simulink model "Sim_HOSMD"  (R2021a)
settings: Solver=VariableStepAuto  StartTime=ti  StopTime=tf  RelTol=1e-3
values from neighbouring files (symbols this model uses):
  a = 2    [InitParams.m]
  k = 1    [InitParams.m]
  omega = 2    [InitParams.m]
undefined symbols (not defined in the file or in its folder): Noise
libraries: simulink x1
settings Model: Creator=perruquetti  LastModifiedBy=perruquetti
settings SolverCC: AlgebraicLoopSolver=TrustRegion
settings DataIOCC: ReturnWorkspaceOutputs=off
settings DebuggingCC: SFMachineParentedDataDiag=warning  ArithmeticOperatorsInVariantConditions=warning
settings SFSimCC: SimUseLocalCustomCode=off  CustomCodeUndefinedFunction=UseInterfaceOnly
settings RTWCC: RTWUseLocalCustomCode=off

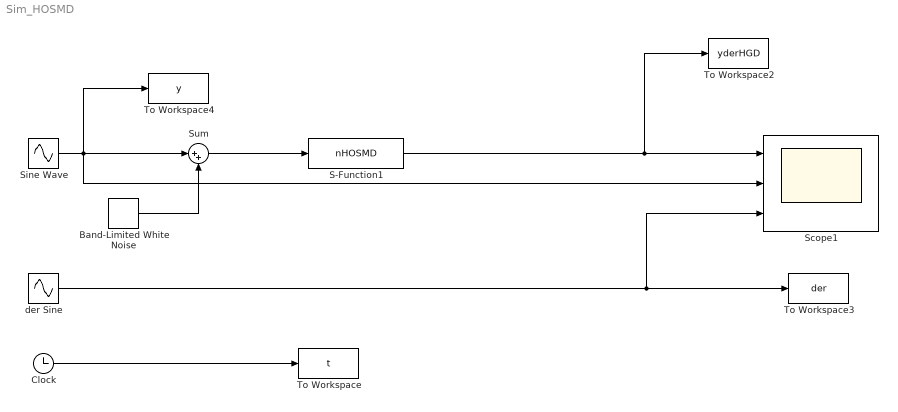
== system Sim_HOSMD ==
  Band-Limited White Noise : simulink/Sources/Band-Limited White Noise  Cov=Noise.power  Ts=Noise.sampling  seed=Noise.seed
  Clock : Clock
  S-Function1 : S-Function  FunctionName=nHOSMD  Parameters=paramsnHOSMD  SFunctionDeploymentMode=off  EnableBusSupport=off
  Scope1 : Scope  NumInputPorts=3
  Sine Wave : Sin  Amplitude=a  Frequency=omega  SampleTime=0
  Sum : Sum  Inputs=|++
  To Workspace : ToWorkspace  VariableName=t  SampleTime=-1
  To Workspace2 : ToWorkspace  VariableName=yderHGD  SampleTime=-1
  To Workspace3 : ToWorkspace  VariableName=der  SampleTime=-1
  To Workspace4 : ToWorkspace  VariableName=y  SampleTime=-1
  der Sine : Sin  Amplitude=a*omega^k  Frequency=omega  Phase=k*pi/2  SampleTime=0
  wires:
  Clock/1 -> To Workspace/1
  Sine Wave/1 -> Scope1/2, Sum/1, To Workspace4/1
  Band-Limited White Noise/1 -> Sum/2
  Sum/1 -> S-Function1/1
  der Sine/1 -> Scope1/3, To Workspace3/1
  S-Function1/1 -> To Workspace2/1, Scope1/1
